simulink model "battery"  (R2022a)
settings: Solver=VariableStepAuto  StartTime=0.0  StopTime=Sim_time  RelTol=1e-3
undefined symbols (not defined in the file): C, I, OCV, R_Discharge, SOC
settings Model: Creator=DDYD  LastModifiedBy=DDYD

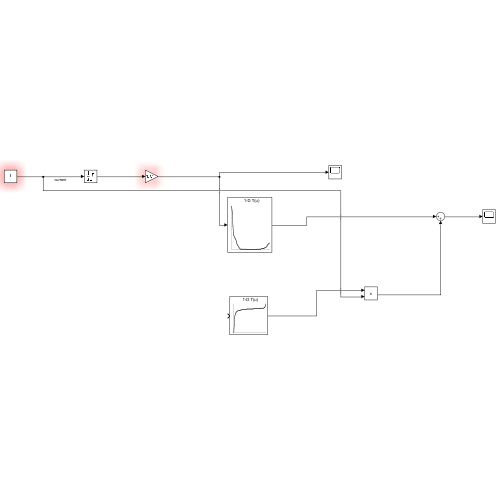
[thumbnail: Simulink's stored preview of the top-level diagram]
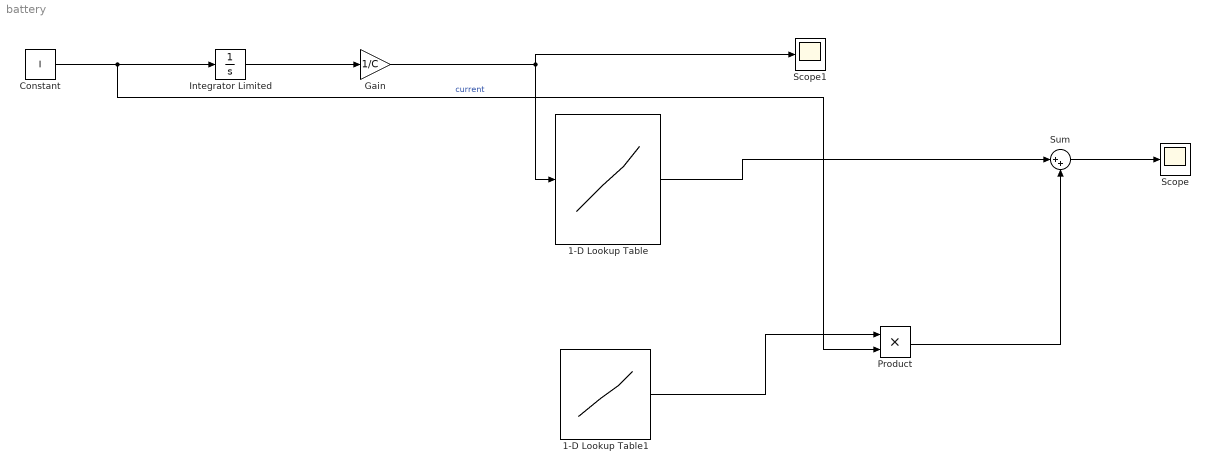
== system battery ==
  1-D Lookup Table : Lookup_n-D  NumberOfTableDimensions=1  BreakpointsForDimension1=SOC  Table=R_Discharge  InternalRulePriority=Speed  RndMeth=Simplest
  1-D Lookup Table1 : Lookup_n-D  NumberOfTableDimensions=1  BreakpointsForDimension1=SOC  Table=OCV  InternalRulePriority=Speed  RndMeth=Simplest
  Constant : Constant  Value=I
  Gain : Gain  Gain=1/C
  Integrator Limited : Integrator  LimitOutput=on  UpperSaturationLimit=1  LowerSaturationLimit=0
  Product : Product
  Scope : Scope
  Scope1 : Scope
  Sum : Sum  Inputs=|++
  wires:
  Constant/1 -> Product/2, Integrator Limited/1  "current"
  Integrator Limited/1 -> Gain/1
  Gain/1 -> Scope1/1, 1-D Lookup Table/1
  1-D Lookup Table1/1 -> Product/1
  Product/1 -> Sum/2
  1-D Lookup Table/1 -> Sum/1
  Sum/1 -> Scope/1
